simulink model "zoh_or_not"  (R2015b)
settings: Solver=FixedStepAuto  StartTime=0.0  StopTime=10.0  RelTol=1e-3
libraries: simulink x2
settings Model: Creator=kjartan  LastModifiedBy=kjartan

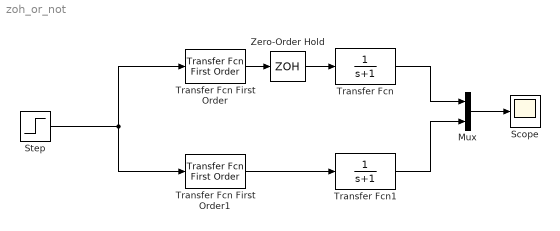
== system zoh_or_not ==
  Mux : Mux  Inputs=2
  Scope : Scope
  Step : Step  SampleTime=1
  Transfer Fcn : TransferFcn  Denominator=[1 1]
  Transfer Fcn First Order : simulink/Discrete/Transfer Fcn First Order  PoleZ=0.7  ICPrevOutput=0.0  DoSatur=off
  Transfer Fcn First Order1 : simulink/Discrete/Transfer Fcn First Order  PoleZ=0.7  ICPrevOutput=0.0  DoSatur=off
  Transfer Fcn1 : TransferFcn  Denominator=[1 1]
  Zero-Order Hold : ZeroOrderHold
  wires:
  Step/1 -> Transfer Fcn First Order/1, Transfer Fcn First Order1/1
  Transfer Fcn First Order/1 -> Zero-Order Hold/1
  Zero-Order Hold/1 -> Transfer Fcn/1
  Transfer Fcn First Order1/1 -> Transfer Fcn1/1
  Transfer Fcn/1 -> Mux/1
  Transfer Fcn1/1 -> Mux/2
  Mux/1 -> Scope/1
